simulink model "SeriesWoundDCMotor"  (R2023a)
settings: Solver=VariableStepAuto  StartTime=0.0  StopTime=1  RelTol=1e-3
values from neighbouring files (symbols this model uses):
  b = 0.001    [Lab1_constants.m]
  Cm = 1.3    [Lab1_constants.m]
  Cw = 3.15    [Lab1_constants.m]
  J = 7*10^(-6)    (= 7e-06)    [Lab1_constants.m]
  La = 0.0015    [Lab1_constants.m]
  Lf = 0.013    [Lab1_constants.m]
  Ra = 8    [Lab1_constants.m]
settings Model: Creator=mikha  LastModifiedBy=mikha

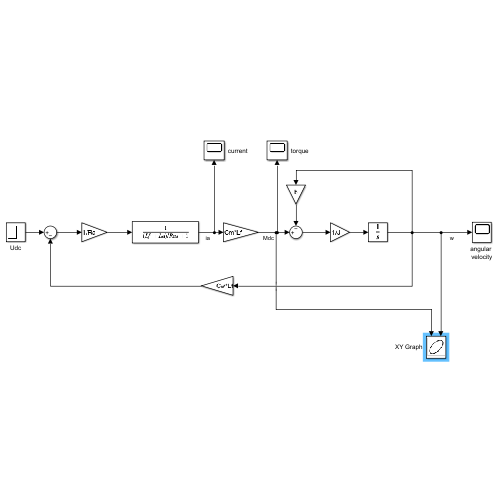
[thumbnail: Simulink's stored preview of the top-level diagram]
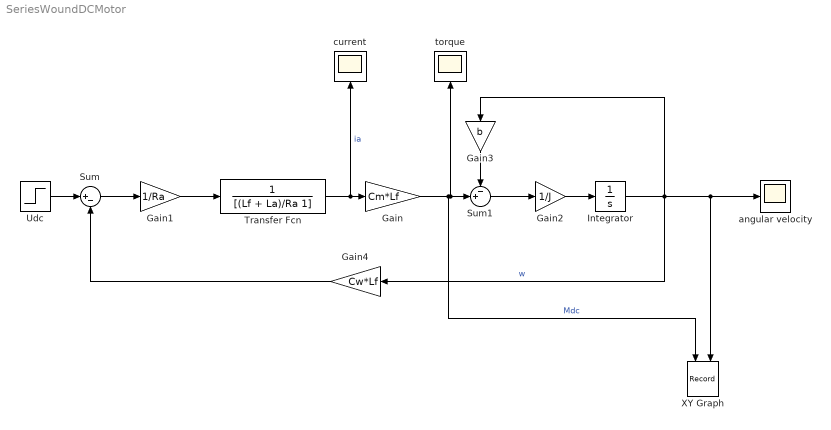
== system SeriesWoundDCMotor ==
  Gain : Gain  Gain=Cm*Lf
  Gain1 : Gain  Gain=1/Ra
  Gain2 : Gain  Gain=1/J
  Gain3 : Gain  Gain=b
  Gain4 : Gain  Gain=Cw*Lf
  Integrator : Integrator
  Sum : Sum  Inputs=|+-
  Sum1 : Sum  Inputs=-+|
  Transfer Fcn : TransferFcn  Denominator=[(Lf + La)/Ra 1]
  Udc : Step  Time=0  After=5  SampleTime=0
  XY Graph : Record  FileSettingsInternal="{\"entries\":[{\"content\":{\"excelSettings\":{\"content\":{},\"type\":\"Streamout.ExcelSettings\"}},\"type\":\"Streamout.FileSettingStorage\",\"uuid\":\"528767e1-7320-42bb-9321-d407354188c7\"}],\"packageUris\":[\"http://schema.mathworks.com/mf0/streamout_blocks/R2020a\"],\"version\":\"1.0\"}"  Layout=[1 1]  SignalsInternal="{\"entries\":[{\"content\":{\"signals\":[{\"content\":{\"blockPath\":[\"SeriesWoundDCMotor/XY Graph\"],\"dimensions\":[1],\"domain\":\"SeriesWoundDCMotor/XY Graph\",\"lineColor\":\"#a2142f\",\"plots\":[1],\"port\":1,\"sid\":[\"\"],\"signalID\":77,\"signalName\":\"Mdc\"},\"type\":\"RecordBlkView.Signal\",\"uuid\":\"6c2de2cb-2da1-48f2-8948-2fb98b1d259b\"},{\"content\":{\"blockPath\":[\"SeriesWoundDCMotor/XY Graph\"],\"dimensions\":[1],\"domain\":\"SeriesWoundDCMotor/XY Graph\",\"lineColor\":\"#139fff\",\"plots\":[1],\"port\":2,\"sid\":[\"\"],\"signalID\":81,\"signalName\":\"w\"},\"type\":\"RecordBlkView.Signal\",\"uuid\":\"ea902109-b696-4175-ae47-ffd1d2ba4d16\"}]},\"type\":\"RecordBlkView.InputSignals\",\"uuid\":\"f719c7e8-85e0-48db-b322-9e4a81c35ad9\"}],\"packageUris\":[\"http://schema.mathworks.com/mf0/streamout_blocks/R2020a\"],\"version\":\"1.0\"}"  VisualizationBindings="{\"xyplotplugin\":{\"info\":[{\"series\":[{\"bindingParametersList\":[{\"parameter\":\"X-Axis\",\"signalID\":81,\"signalName\":\"w\"},{\"parameter\":\"Y-Axis\",\"signalID\":77,\"signalName\":\"Mdc\"}],\"seriesID\":37869}],\"subplotID\":1}]}}"  CompatibilityTag=XY
  angular velocity : Scope
  current : Scope
  torque : Scope
  wires:
  Udc/1 -> Sum/1
  Sum/1 -> Gain1/1
  Transfer Fcn/1 -> current/1, Gain/1  "ia"
  Gain/1 -> XY Graph/1, torque/1, Sum1/2  "Mdc"
  Sum1/1 -> Gain2/1
  Gain2/1 -> Integrator/1
  Gain3/1 -> Sum1/1
  Gain1/1 -> Transfer Fcn/1
  Gain4/1 -> Sum/2
  Integrator/1 -> XY Graph/2, angular velocity/1, Gain3/1, Gain4/1  "w"
